simulink model "Trafficlight"  (R2021a)
settings: Solver=FixedStepAuto  StartTime=0.0  StopTime=20  FixedStep=3  RelTol=1e-3
settings Model: Creator=Ms store  LastModifiedBy=Ms store

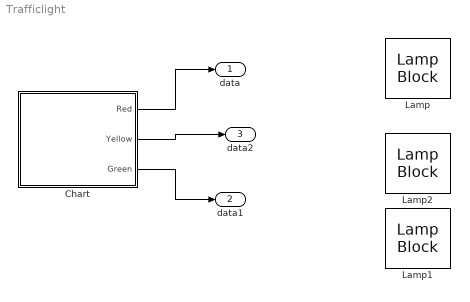
== system Trafficlight ==
  Chart : Stateflow chart  TreatAsAtomicUnit=on
  Lamp : LampBlock
  Lamp1 : LampBlock
  Lamp2 : LampBlock
  data : Outport
  data1 : Outport  Port=2
  data2 : Outport  Port=3
  wires:
  Chart/1(Red) -> data/1
  Chart/3(Green) -> data1/1
  Chart/2(Yellow) -> data2/1

== stateflow chart Trafficlight/Chart ==
  state Stop
    Red=1;
    Yellow=0;
    Green=0;
  state Ready
    Red=0;
    Yellow=1;
    Green=0;
  state Go
    Red=0;
    Yellow=0;
    Green=1;
  (default) -> Stop
  Go -> Stop : [after(3,tick)]
  Stop -> Ready : [after(3,tick)]
  Ready -> Go : [after(3,tick)]
  data: Red output; Yellow output; Green output
